simulink model "Signal_Conversion_Bus"  (R2014a)
settings: Solver=FixedStepDiscrete  StartTime=0.0  StopTime=10.0  FixedStep=0.1  RelTol=1e-3
settings Model: BufferReuse=off  Creator=kohei-y  LastModifiedBy=ts1413
settings DataIOCC: SaveOutput=off
settings OptimizationCC: BlockReduction=off  OptimizeBlockIOStorage=off  BufferReuse=off  GlobalBufferReuse=off  ExpressionFolding=off  LocalBlockOutputs=off  OptimizeModelRefInitCode=on  LifeSpan=1
settings RTWCC: SystemTargetFile=ert.tlc  GenCodeOnly=on  TemplateMakefile=ert_default_tmf  Description=Embedded Coder  ProcessScript=ert_make_rtw_hook  IncludeHyperlinkInReport=on
settings CodeAppCC: IgnoreCustomStorageClasses=off
settings ERTTargetCC: ParMdlRefBuildCompliant=on  CompOptLevelCompliant=on  ConcurrentExecutionCompliant=on  ERTFirstTimeCompliant=on  ModelStepFunctionPrototypeControlCompliant=on  CPPClassGenCompliant=on  InlinedParameterPlacement=Hierarchical  ERTCustomFileTemplate=example_file_process.tlc

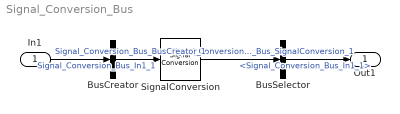
== system Signal_Conversion_Bus ==
  In1 : Inport
  BusCreator : BusCreator  Inputs=1  OutDataTypeStr=Bus: BusObject
  BusSelector : BusSelector  OutputSignals=Signal_Conversion_Bus_In1_1
  SignalConversion : SignalConversion  ConversionOutput=Nonvirtual bus
  Out1 : Outport
  wires:
  SignalConversion/1 -> BusSelector/1  "Signal_Conversion_Bus_SignalConversion_1"
  In1/1 -> BusCreator/1  "Signal_Conversion_Bus_In1_1"
  BusCreator/1 -> SignalConversion/1  "Signal_Conversion_Bus_BusCreator_1"
  BusSelector/1 -> Out1/1  "<Signal_Conversion_Bus_In1_1>"
